simulink model "test_pos_ctrl_target"  (R2014a)
settings: Solver=ode5  StartTime=0.0  StopTime=inf  FixedStep=basic_time_step  RelTol=1e-3
values from neighbouring files (symbols this model uses):
  basic_time_step = 0.002    [init_pos_ctrl_target.m]
  g = 9.81    [init_pos_ctrl_target.m]
  kd = [2 0 0 ... (first row only)    [init_pos_ctrl_target.m]
  KDP = 11/5    (= 2.2)    [init_pos_ctrl_target.m]
  KDR = 11/5    (= 2.2)    [init_pos_ctrl_target.m]
  KDY = 11    [init_pos_ctrl_target.m]
  ki = 0*[.1 0 0 ... (first row only)    [init_pos_ctrl_target.m]
  kp = [1 0 0 ... (first row only)    [init_pos_ctrl_target.m]
  KPP = 30/5    (= 6)    [init_pos_ctrl_target.m]
  KPR = 30/5    (= 6)    [init_pos_ctrl_target.m]
  KPY = 30    [init_pos_ctrl_target.m]
  m0 = 1.3    [init_pos_ctrl_target.m]
  max_pitch = sin(15*pi/180)    [init_pos_ctrl_target.m]
  max_roll = sin(15*pi/180)    [init_pos_ctrl_target.m]
undefined symbols (not defined in the file or in its folder): DiscIntNeverNeededParam, IMU_time_step, VICON_time_step
libraries: geometry_msgs x3, sensor_msgs x1, rt_sync x1
settings Model: Creator=prg  LastModifiedBy=fschiano
settings OptimizationCC: ExpressionDepthLimit=2147483647
settings DebuggingCC: UnderspecifiedInitializationDetection=Classic  StateNameClashWarn=warning

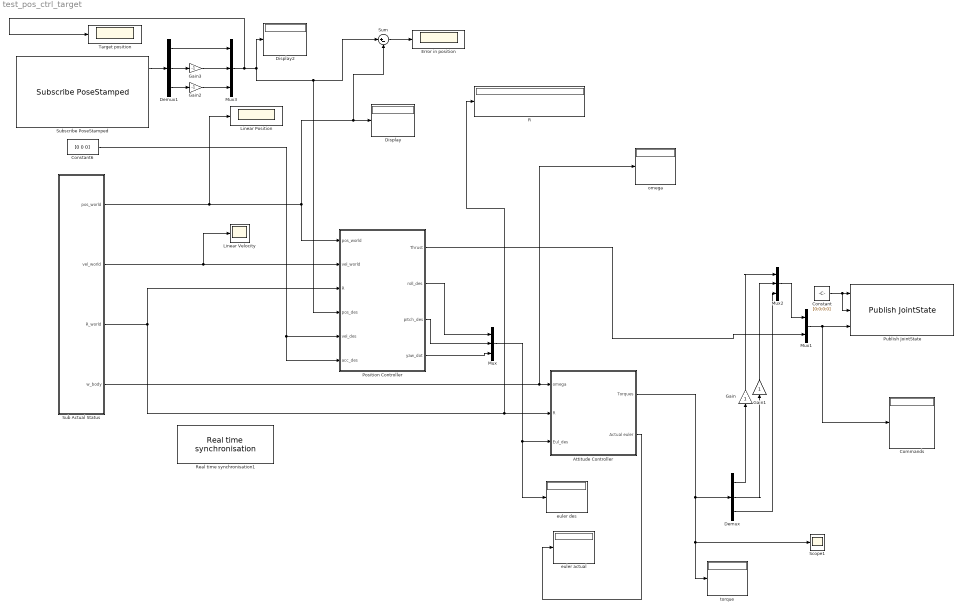
== system test_pos_ctrl_target ==
  " R" : Display
  Attitude Controller : Subsystem  SystemSampleTime=IMU_time_step
  Commands : Display
  Constant : Constant  Value=[0;0;0;0]
  Constant6 : Constant  Value=[0 0 0]
  Demux : Demux  Outputs=3
  Demux1 : Demux  Outputs=3
  Display : Display
  Display2 : Display
  Error in position : Scope
      settings: TimeRange=10  YMin=-4  YMax=7.5
  Gain : Gain
  Gain1 : Gain
  Gain2 : Gain  Gain=-1
  Gain3 : Gain  Gain=-1
  Linear Position : Scope
      settings: YMin=-4.25  YMax=0.25  SaveName=ScopeData2
  Linear Velocity : Scope
      settings: YMin=-0.8  YMax=0.6  SaveName=ScopeData3
  Mux : Mux  Inputs=3
  Mux1 : Mux  Inputs=2
  Mux2 : Mux  Inputs=3
  Mux3 : Mux  Inputs=3
  Position Controller : Subsystem  SystemSampleTime=VICON_time_step
  Publish JointState : sensor_msgs/Publish JointState  stepTime=basic_time_step  topic_prefix='/command/quadrotor_'  list_of_robot_ids=char([0])  topic_postfix=''  n_dofs=char(4)
  Real time synchronisation1 : rt_sync/Real time synchronisation  stepTime=basic_time_step  minShownDelay=0.5  ShowEveryNumCycles=1/basic_time_step  slowDownFactor=1
  Scope1 : Scope
  Sub Actual Status : Subsystem
  Subscribe PoseStamped : geometry_msgs/Subscribe PoseStamped  stepTime=basic_time_step  topic_prefix='/vrep/Quadricopter_target_'  list_of_robot_ids=char([0])  topic_postfix='/pose'
  Sum : Sum  Inputs=|+-
  Target position : Scope
      settings: YMin=-4  YMax=0.25  SaveName=ScopeData4
  euler actual : Display
  euler des : Display
  omega : Display
  "torque " : Display
  wires:
  Constant6/1 -> Position Controller/6(acc_des), Position Controller/5(vel_des)
  Position Controller/2(roll_des) -> Mux/1
  Mux/1 -> euler des/1, Attitude Controller/3(Eul_des)
  Position Controller/3(pitch_des) -> Mux/2
  Position Controller/4(yaw_dot) -> Mux/3
  Mux1/1 -> Commands/1, Publish JointState/3
  Constant/1 -> Publish JointState/2, Publish JointState/1
  Position Controller/1(Thrust) -> Mux1/2
  Sub Actual Status/1(pos_world) -> Linear Position/1, Sum/2, Display/1, Position Controller/1(pos_world)
  Sub Actual Status/2(vel_world) -> Linear Velocity/1, Position Controller/2(vel_world)
  Sub Actual Status/4(w_body) -> omega/1, Attitude Controller/1(omega)
  Attitude Controller/1(Torques) -> Demux/1, Scope1/1, "torque "/1
  Sub Actual Status/3("R_world ") -> " R"/1, Attitude Controller/2(R), Position Controller/3(R)
  Attitude Controller/2(Actual euler) -> euler actual/1
  Demux/3 -> Mux2/3
  Mux2/1 -> Mux1/1
  Demux/1 -> Gain/1
  Demux/2 -> Gain1/1
  Gain/1 -> Mux2/1
  Gain1/1 -> Mux2/2
  Subscribe PoseStamped/1 -> Demux1/1
  Mux3/1 -> Display2/1, Sum/1, Position Controller/4(pos_des), Target position/1
  Demux1/2 -> Gain3/1
  Demux1/1 -> Mux3/1
  Demux1/3 -> Gain2/1
  Gain2/1 -> Mux3/3
  Gain3/1 -> Mux3/2
  Sum/1 -> Error in position/1

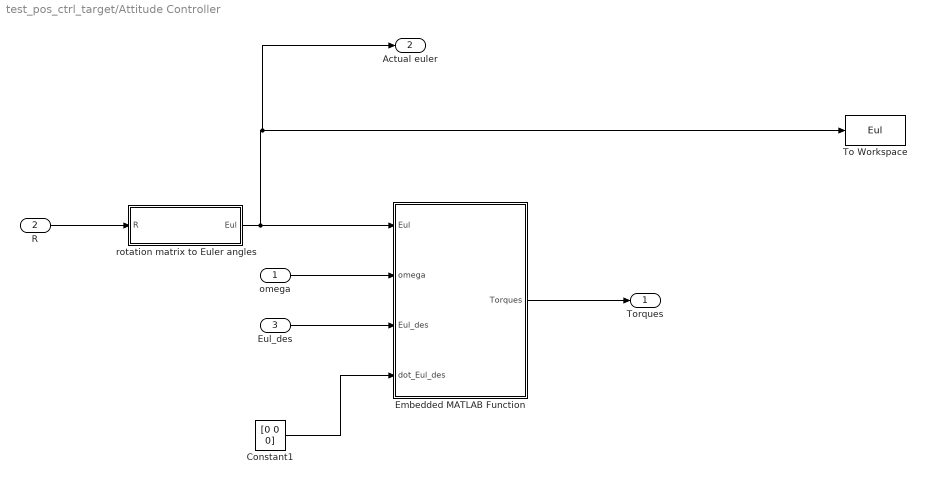
== system test_pos_ctrl_target/Attitude Controller ==
  omega : Inport
  R : Inport  Port=2
  Eul_des : Inport  Port=3
  Constant1 : Constant  Value=[0 0 0]
  Embedded MATLAB Function : MATLAB Function  TreatAsAtomicUnit=on
  To Workspace : ToWorkspace  VariableName=Eul  SampleTime=-1
  rotation matrix to Euler angles : MATLAB Function  TreatAsAtomicUnit=on
  Torques : Outport
  Actual euler : Outport  Port=2
  wires:
  R/1 -> rotation matrix to Euler angles/1(R)
  rotation matrix to Euler angles/1(Eul) -> Embedded MATLAB Function/1(Eul), Actual euler/1, To Workspace/1
  omega/1 -> Embedded MATLAB Function/2(omega)
  Eul_des/1 -> Embedded MATLAB Function/3(Eul_des)
  Embedded MATLAB Function/1(Torques) -> Torques/1
  Constant1/1 -> Embedded MATLAB Function/4(dot_Eul_des)

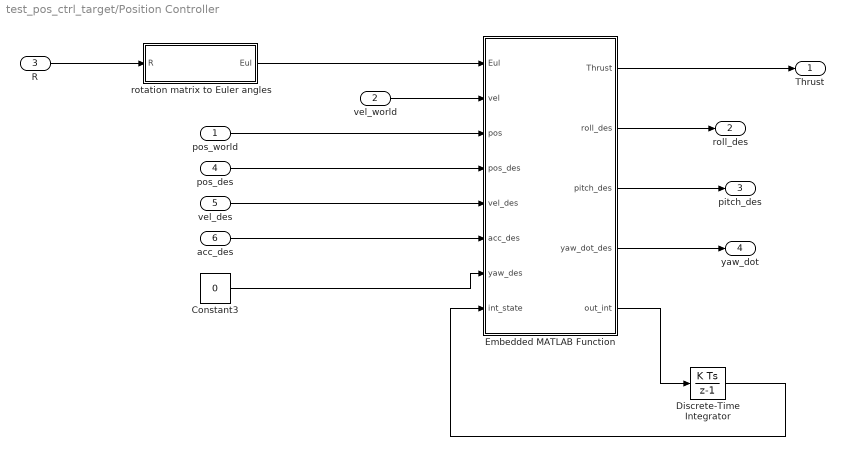
== system test_pos_ctrl_target/Position Controller ==
  pos_world : Inport
  vel_world : Inport  Port=2
  R : Inport  Port=3
  pos_des : Inport  Port=4
  vel_des : Inport  Port=5
  acc_des : Inport  Port=6
  Constant3 : Constant  Value=0
  Discrete-Time Integrator : DiscreteIntegrator  InitialCondition=[0 0 0]  SampleTime=-1  ICPrevOutput=DiscIntNeverNeededParam  ICPrevScaledInput=DiscIntNeverNeededParam
  Embedded MATLAB Function : MATLAB Function  TreatAsAtomicUnit=on
  rotation matrix to Euler angles : MATLAB Function  TreatAsAtomicUnit=on
  Thrust : Outport
  roll_des : Outport  Port=2
  pitch_des : Outport  Port=3
  yaw_dot : Outport  Port=4
  wires:
  R/1 -> rotation matrix to Euler angles/1(R)
  rotation matrix to Euler angles/1(Eul) -> Embedded MATLAB Function/1(Eul)
  vel_world/1 -> Embedded MATLAB Function/2(vel)
  pos_world/1 -> Embedded MATLAB Function/3(pos)
  Embedded MATLAB Function/1(Thrust) -> Thrust/1
  pos_des/1 -> Embedded MATLAB Function/4(pos_des)
  vel_des/1 -> Embedded MATLAB Function/5(vel_des)
  acc_des/1 -> Embedded MATLAB Function/6(acc_des)
  Constant3/1 -> Embedded MATLAB Function/7(yaw_des)
  Embedded MATLAB Function/2(roll_des) -> roll_des/1
  Embedded MATLAB Function/3(pitch_des) -> pitch_des/1
  Embedded MATLAB Function/4(yaw_dot_des) -> yaw_dot/1
  Embedded MATLAB Function/5(out_int) -> Discrete-Time Integrator/1
  Discrete-Time Integrator/1 -> Embedded MATLAB Function/8(int_state)

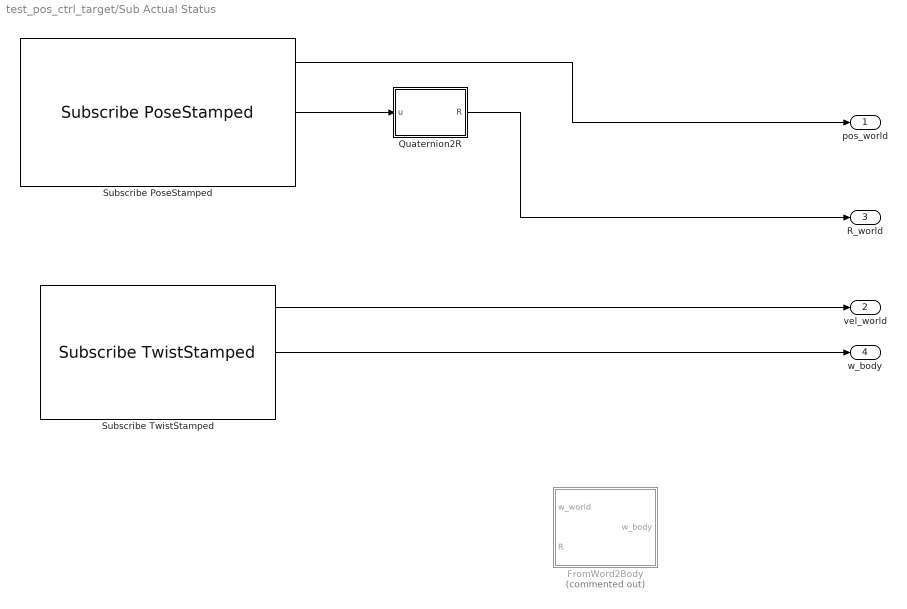
== system test_pos_ctrl_target/Sub Actual Status ==
  FromWord2Body : MATLAB Function  Commented=on  TreatAsAtomicUnit=on
  Quaternion2R : MATLAB Function  TreatAsAtomicUnit=on
  Subscribe PoseStamped : geometry_msgs/Subscribe PoseStamped  stepTime=basic_time_step  topic_prefix='/vrep/pose/quadrotor_'  list_of_robot_ids=char([0])  topic_postfix=''
  Subscribe TwistStamped : geometry_msgs/Subscribe TwistStamped  stepTime=basic_time_step  topic_prefix='/vrep/twist/quadrotor_'  list_of_robot_ids=char([0])  topic_postfix=''
  pos_world : Outport
  vel_world : Outport  Port=2
  "R_world " : Outport  Port=3
  w_body : Outport  Port=4
  wires:
  Subscribe PoseStamped/1 -> pos_world/1
  Subscribe PoseStamped/2 -> Quaternion2R/1(u)
  Quaternion2R/1(R) -> "R_world "/1
  Subscribe TwistStamped/1 -> vel_world/1
  Subscribe TwistStamped/2 -> w_body/1

== matlab function test_pos_ctrl_target/Attitude Controller/Embedded MATLAB Function ==
  data: Eul input; Torques output; omega input; Eul_des input; dot_Eul_des input; KDR parameter; KPR parameter; KDP parameter; KPP parameter; KDY parameter; KPY parameter
function Torques  = fcn(Eul, omega, Eul_des, dot_Eul_des, KDR, KPR, KDP, KPP, KDY, KPY)
% This block supports the Embedded MATLAB subset.
% See the help menu for details. 

% p = angles(2);
% r = angles(1);
% y=angles(3);
% 
% T = [1      tan(p)*sin(r) tan(p)*cos(r);
%     0       cos(r)  -sin(r);
%     0       sin(r)/cos(p)   cos(r)/cos(p)];
% 
% dot_ang = T*omega;
% dot_r=dot_ang(1);
% dot_p = dot_ang(2);
% 
% T_dot = [0  tan(p)*cos(r)*dot_r+(sin(r)+tan(p)^2*sin(r))*dot_p -tan(p)*sin(r)*dot_r+(cos(r)+tan(p)^2*cos(r))*dot_p;
%          0  -sin(r)*dot_r   -cos(r)*dot_r;
%          0  cos(r)/cos(p)*dot_r+sin(r)*sin(p)/cos(p)^2*dot_p    -sin(r)/cos(p)*dot_r+cos(r)*sin(p)/cos(p)^2*dot_p];
% 
% 
% k_d = 11;
% k_p = 30;
% ang_vel_des = [0 0 yaw_dot_des]';
% 
% 
% if(yaw_des - angles(3) > pi)
%     angles(3) = angles(3)+2*pi;
% elseif (yaw_des - angles(3) < -pi)
%     angles(3) = angles(3)-2*pi;
% end
% 
% ang_des = [roll_des pitch_des yaw_des]';
% U = I*inv(T)*(k_d*(ang_vel_des-dot_ang)+k_p*(ang_des - angles)-T_dot*omega)+cross(omega, I*omega);
% r_c = U(1);
% p_c = U(2);
% y_c = U(3);

Torques=[0;0;0];

r = Eul(1);
p = Eul(2);
y = Eul(3);




T = [1      tan(p)*sin(r) tan(p)*cos(r);
    0       cos(r)  -sin(r);
    0       sin(r)/cos(p)   cos(r)/cos(p)];


% T=eye(3);

dot_Eul = T*omega;

dot_r = dot_Eul(1);
dot_p = dot_Eul(2);
dot_y = dot_Eul(3);

% U=I*inv(T)*([ KDR * (0 - dot_r) + KPR * (roll_des - r); KDP * (0 - dot_p) + KPP * (pitch_des - p) ; KPY * (yaw_dot_des - dot_y) ]);


Torques(1) = KDR * (dot_Eul_des(1) - dot_r) + KPR * (Eul_des(1) - r);
Torques(2) = KDP * (dot_Eul_des(2) - dot_p) + KPP * (Eul_des(2) - p);
Torques(3) = KDY * (dot_Eul_des(3) - dot_y) + KPY * (Eul_des(3) - y);


% if abs(Torques(1)) > 0.02
%     Torques(1)= 0.02;
%     
% end
% 
% 
% if abs(Torques(2)) > 0.02
%     Torques(2)= 0.02;
%     
% end

== matlab function test_pos_ctrl_target/Sub Actual Status/Quaternion2R ==
  data: u input; R output
function R = fcn(u)


   



w = u( 1 );
x = u( 2 );
y = u( 3 );
z = u( 4 );

n = sqrt(x*x + y*y + z*z + w*w);


    x = x/ n;
    y = y/ n;
    z = z/ n;
    w = w/ n;

Rxx = 1 - 2*(y^2 + z^2);
Rxy = 2*(x*y - z*w);
Rxz = 2*(x*z + y*w);

Ryx = 2*(x*y + z*w);
Ryy = 1 - 2*(x^2 + z^2);
Ryz = 2*(y*z - x*w );

Rzx = 2*(x*z - y*w );
Rzy = 2*(y*z + x*w );
Rzz = 1 - 2 *(x^2 + y^2);

R = [ 
    Rxx,    Rxy,    Rxz;
    Ryx,    Ryy,    Ryz;
    Rzx,    Rzy,    Rzz];

% 
% 
% a = u( 1 );
% b = u( 2 );
% c = u( 3 );
% d = u( 4 );
% 
% 
%   R(1,1) = a*a+b*b-c*c-d*d;
%   R(1,2) = 2*b*c-2*a*d;
%   R(1,3) = 2*a*c+2*b*d;
%   
%   R(2,1)   = 2*a*d+2*b*c;
%   R(2,2)  = a*a-b*b+c*c-d*d;
%   R(2,3)  = 2*c*d-2*a*b;
%    
%   R(3,1)    = 2*b*d-2*a*c;
%   R(3,2)    = 2*a*b+2*c*d;
%   R(3,3)    = a*a-b*b-c*c+d*d;
% 
%

== matlab function test_pos_ctrl_target/Position Controller/Embedded MATLAB Function ==
  data: Eul input; Thrust output; roll_des output; pitch_des output; yaw_dot_des output; vel input; pos input; pos_des input; vel_des input; acc_des input; yaw_des input; int_state input; m0 parameter; g parameter; out_int output; kd parameter; kp parameter; ki parameter; max_roll parameter; max_pitch parameter
function [Thrust, roll_des, pitch_des, yaw_dot_des, out_int]  = fcn(Eul, vel, pos, pos_des, vel_des, acc_des, yaw_des, int_state, m0, g, kd, kp, ki, max_roll, max_pitch)
% This block supports the Embedded MATLAB subset
% See the help menu for details. 


r = Eul(1);
p = Eul(2);
y = Eul(3);



Thrust=m0/(cos(r)*cos(p))*(-g + acc_des(3) + kd(3,3)*(vel_des(3) -vel(3)) + kp(3,3)*(pos_des(3)-pos(3)) + int_state(3) );


out_int=ki*(pos_des-pos);



% max_T=30;
% 
% if abs(T(3))>max_T
%     T(3)=sign(T(3))*max_T;
% end

if (Thrust>-5)
    Thrust=-5;
end


if (Thrust<-2*m0*g+5)
    Thrust=-2*m0*g+5;
end




% roll_des=-m/T(3)*( acc_des(2) + kd*(vel_des(2) -vel(2)) + kp*(pos_des(2)-pos(2)) );
% pitch_des=m/T(3)*( acc_des(1) + kd*(vel_des(1) -vel(1)) + kp*(pos_des(1)-pos(1)) );


ddpx=kd(1,1)*(vel_des(1) -vel(1)) + kp(1,1)*(pos_des(1)-pos(1) + int_state(1) );
ddpy=kd(2,2)*(vel_des(2) -vel(2)) + kp(2,2)*(pos_des(2)-pos(2) + int_state(2) );



ctrl_roll=m0/Thrust*( -sin(y)*ddpx+cos(y)*ddpy);

if abs(ctrl_roll)>max_roll
    ctrl_roll=sign(ctrl_roll)*max_roll;
end

ctrl_pitch= m0/(Thrust*cos(r))*( cos(y)*ddpx+sin(y)*ddpy);


if abs(ctrl_pitch)>max_pitch
    ctrl_pitch=sign(ctrl_pitch)*max_pitch;
end





roll_des = -asin( ctrl_roll );

pitch_des = asin(  ctrl_pitch );

yaw_dot_des = 0; % kp(3,3)*(yaw_des-y);

== matlab function test_pos_ctrl_target/Position Controller/rotation matrix to Euler angles ==
  data: R input; Eul output
function Eul = eulerangles(R)
% This block supports an embeddable subset of the MATLAB language.
% See the help menu for details. 

Roll = atan2(R(3,2),R(3,3));
Pitch = atan2(-R(3,1),sqrt(R(3,2)^2+R(3,3)^2));
Yaw = atan2(R(2,1),R(1,1));


Eul = [Roll; Pitch; Yaw];

== matlab function test_pos_ctrl_target/Sub Actual Status/FromWord2Body ==
  data: w_world input; w_body output; R input
function w_body = fcn(w_world,R)




w_body = R * w_world;

== matlab function test_pos_ctrl_target/Attitude Controller/rotation matrix to Euler angles ==
  data: R input; Eul output
function Eul = eulerangles(R)
% This block supports an embeddable subset of the MATLAB language.
% See the help menu for details. 

Roll = atan2(R(3,2),R(3,3));
Pitch = atan2(-R(3,1),sqrt(R(3,2)^2+R(3,3)^2));
Yaw = atan2(R(2,1),R(1,1));


Eul = [Roll; Pitch; Yaw];
